simulink model "SOlar_panel_project"  (R2023b)
settings: Solver=FixedStepDiscrete  StartTime=0.0  StopTime=inf  FixedStep=1e-3  RelTol=1e-3
settings Model: ExtModeTrigDuration=2  Creator=Beshary  LastModifiedBy=Beshary
settings OptimizationCC: DefaultParameterBehavior=Inlined  UseDivisionForNetSlopeComputation=on  GainParamInheritBuiltInType=on  UseFloatMulNetSlope=on  InlineInvariantSignals=on  PassReuseOutputArgsAs=Individual arguments  ZeroExternalMemoryAtStartup=off  ZeroInternalMemoryAtStartup=off  NoFixptDivByZeroProtection=on  EfficientFloat2IntCast=on  LifeSpan=1  MaxStackSize=64  OptimizeBlockOrder=speed  DifferentSizesBufferReuse=on  EfficientTunableParamExpr=on
settings DebuggingCC: ParameterTunabilityLossMsg=error
settings HardwareCC: ProdBitPerInt=16  ProdBitPerPointer=16  ProdBitPerSizeT=16  ProdBitPerPtrDiffT=16  ProdLargestAtomicFloat=None  ProdWordSize=8  ProdLongLongMode=on  ProdHWDeviceType=Atmel->AVR
settings SFSimCC: MATLABDynamicMemAlloc=off
settings RTWCC: Description=Embedded Coder  SystemTargetFile=ert.tlc  HardwareBoard=Arduino Uno  TemplateMakefile=ert_default_tmf  Toolchain=Arduino AVR  BuildConfiguration=Faster Runs
settings CodeAppCC: ForceParamTrailComments=on  IgnoreCustomStorageClasses=off  OperatorAnnotations=on  SimulinkDataObjDesc=on  SFDataObjDesc=on  CustomSymbolStrGlobalVar=rt$N$M  CustomSymbolStrType=$N$M  CustomSymbolStrFcn=$N$M$F  CustomSymbolStrMacro=$N$M  InsertBlockDesc=on
settings ERTTargetCC: IncludeMdlTerminateFcn=off  CombineSignalStateStructs=on  SupportAbsoluteTime=off  SupportComplex=off  SupportNonInlinedSFcns=on  ExtModeTransport=3  ExtModeStaticAlloc=on  ExtModeAutomaticAllocSize=off  ExtModeStaticAllocSize=250  ExtModeMexFile=ext_xcp  ExtModeIntrfLevel=Level2 - Open  InlinedParameterPlacement=NonHierarchical  ERTFilePackagingFormat=CompactWithDataFile

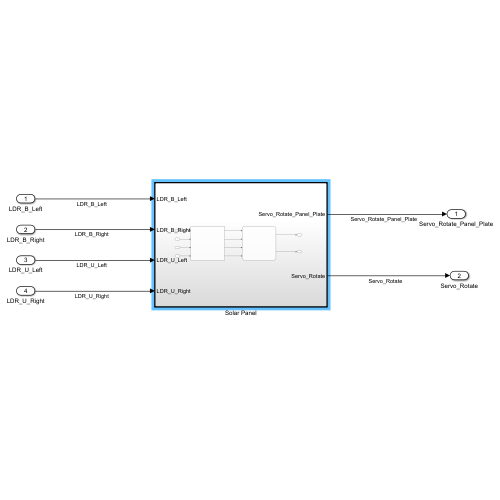
[thumbnail: Simulink's stored preview of the top-level diagram]
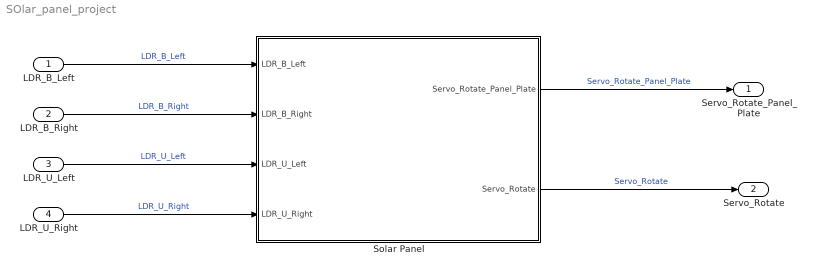
== system SOlar_panel_project ==
  LDR_B_Left : Inport
  LDR_B_Right : Inport  Port=2
  LDR_U_Left : Inport  Port=3
  LDR_U_Right : Inport  Port=4
  Solar Panel : Subsystem  TreatAsAtomicUnit=on
  Servo_Rotate_Panel_Plate : Outport
  Servo_Rotate : Outport  Port=2
  wires:
  LDR_B_Left/1 -> Solar Panel/1(LDR_B_Left)  "LDR_B_Left"
  LDR_B_Right/1 -> Solar Panel/2(LDR_B_Right)  "LDR_B_Right"
  LDR_U_Left/1 -> Solar Panel/3(LDR_U_Left)  "LDR_U_Left"
  LDR_U_Right/1 -> Solar Panel/4(LDR_U_Right)  "LDR_U_Right"
  Solar Panel/1(Servo_Rotate_Panel_Plate) -> Servo_Rotate_Panel_Plate/1  "Servo_Rotate_Panel_Plate"
  Solar Panel/2(Servo_Rotate) -> Servo_Rotate/1  "Servo_Rotate"

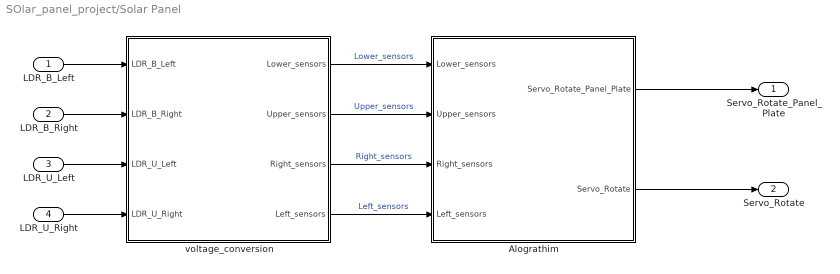
== system SOlar_panel_project/Solar Panel ==
  LDR_B_Left : Inport
  LDR_B_Right : Inport  Port=2
  LDR_U_Left : Inport  Port=3
  LDR_U_Right : Inport  Port=4
  "Alograthim " : Stateflow chart  TreatAsAtomicUnit=on
      settings: PortSchema="{\"entries\":[{\"content\":{\"sides\":[{\"content\":{\"connectorIds\":[\"In2\",\"In1\",\"In3\",\"In4\"]},\"type\":\"ConnectorPlacement.EquallySpacedRectSide\",\"uuid\":\"47346178-62f1-4af9-966f-6088c34d7d3a\"},{\"content\":{\"connectorIds\":[\"Out1\",\"Out2\"],\"side\":\"RIGHT\"},\"type\":\"ConnectorPlacement.EquallySpacedRectSide\",\"uuid\":\"d42f0d69-c7c6-440d-b039-ff859220b6c7\"},{\"content\":{\"side\":\"TOP\"},\"type\":\"ConnectorPlacement.EquallySpacedRectSide\",\"uuid\":\"40083903-8935-43d1-87ca-0c4b4a5851ce\"}]},\"type\":\"ConnectorPlacement.EquallySpacedConnector\",\"uuid\":\"c94df97a-4768-4a21-83be-24c93ffa522d\"}],\"packageUris\":[\"http://schema.mathworks.com/mf0/Connector/R2020b\"],\"version\":\"1.0\"}"
  voltage_conversion : Subsystem
  Servo_Rotate_Panel_Plate : Outport
  Servo_Rotate : Outport  Port=2
  wires:
  voltage_conversion/2(Upper_sensors) -> "Alograthim "/1(Upper_sensors)  "Upper_sensors"
  voltage_conversion/3(Right_sensors) -> "Alograthim "/3(Right_sensors)  "Right_sensors"
  LDR_B_Right/1 -> voltage_conversion/2(LDR_B_Right)
  "Alograthim "/2(Servo_Rotate) -> Servo_Rotate/1
  voltage_conversion/1(Lower_sensors) -> "Alograthim "/2(Lower_sensors)  "Lower_sensors"
  LDR_B_Left/1 -> voltage_conversion/1(LDR_B_Left)
  LDR_U_Left/1 -> voltage_conversion/3(LDR_U_Left)
  voltage_conversion/4(Left_sensors) -> "Alograthim "/4(Left_sensors)  "Left_sensors"
  "Alograthim "/1(Servo_Rotate_Panel_Plate) -> Servo_Rotate_Panel_Plate/1
  LDR_U_Right/1 -> voltage_conversion/4(LDR_U_Right)

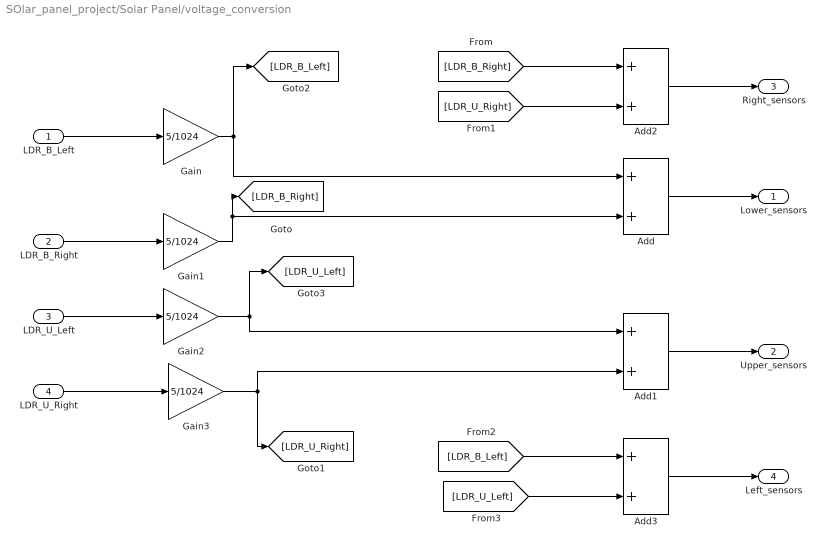
== system SOlar_panel_project/Solar Panel/voltage_conversion ==
  LDR_B_Left : Inport
  LDR_B_Right : Inport  Port=2
  LDR_U_Left : Inport  Port=3
  LDR_U_Right : Inport  Port=4
  Add{,1..3} (4 alike) : Sum
  Gain{,1..3} (4 alike) : Gain  Gain=5/1024
  Lower_sensors : Outport
  Upper_sensors : Outport  Port=2
  Right_sensors : Outport  Port=3
  Left_sensors : Outport  Port=4
  wires:
  LDR_U_Right/1 -> Gain3/1
  LDR_U_Left/1 -> Gain2/1
  LDR_B_Right/1 -> Gain1/1
  LDR_B_Left/1 -> Gain/1
  Gain3/1 -> [LDR_U_Right], Add1/2
  Gain/1 -> [LDR_B_Left], Add/1
  Gain1/1 -> [LDR_B_Right], Add/2
  Add/1 -> Lower_sensors/1
  Add1/1 -> Upper_sensors/1
  [LDR_B_Right] -> Add2/1
  [LDR_U_Right] -> Add2/2
  Add2/1 -> Right_sensors/1
  [LDR_B_Left] -> Add3/1
  Add3/1 -> Left_sensors/1
  [LDR_U_Left] -> Add3/2
  Gain2/1 -> [LDR_U_Left], Add1/1

== stateflow chart SOlar_panel_project/Solar Panel/Alograthim  ==
  state Servo_land [parallel]
    en:
    du:
    Servo_Rotate=servo_land(Right_sensors,Left_sensors);
    settings: executionOrder=1
  state servo_panel1 [parallel]
    en:
    du:
    Servo_Rotate_Panel_Plate=servo_panel(Upper_sensors,Lower_sensors);
    settings: executionOrder=2
  state Servo_out=servo_panel(Upper_sensors,Lower_sensors) [function]
    (default) -> (junction 107) : /* speed */
    (junction 107) -> (junction 124) [order 1] : [abs(Upper_sensors-Lower_sensors)<=0.5]
    (junction 107) -> (junction 116) [order 2]
    (junction 124) -> (junction 114) : {Servo_out=0;}
    (junction 116) -> (junction 115) [order 1] : [Upper_sensors>Lower_sensors]
    (junction 116) -> (junction 111) [order 2] : {Servo_out=(Upper_sensors/2)*(255/5)*Step_angle;}
    (junction 115) -> (junction 123) : {Servo_out=(Lower_sensors/2)*(255/5)*Step_angle;}
    (junction 123) -> (junction 111)
    (junction 114) -> (junction 123)
    (junction 111) -> (junction 110)
  state Servo_out_land=servo_land(Right_sensors,Left_sensors) [function]
    (default) -> (junction 99) : /* speed */
    (junction 99) -> (junction 100) [order 1] : [abs(Right_sensors-Left_sensors)<=0.5]
    (junction 99) -> (junction 101) [order 2]
    (junction 100) -> (junction 105) : {Servo_out_land=0;}
    (junction 101) -> (junction 102) [order 1] : [Right_sensors>Left_sensors]
    (junction 101) -> (junction 103) [order 2] : {Servo_out_land=(Right_sensors/2)*(255/5)*Step_angle;}
    (junction 102) -> (junction 104) : {Servo_out_land=(Left_sensors/2)*(255/5)*Step_angle;}
    (junction 104) -> (junction 103)
    (junction 105) -> (junction 104)
    (junction 103) -> (junction 106)
  data: Servo_out function_output double; Upper_sensors function_input double; Lower_sensors function_input double; Servo_out_land function_output double; Right_sensors function_input double; Left_sensors function_input double; Servo_Rotate_Panel_Plate output; Upper_sensors input; Lower_sensors input; Right_sensors input; Left_sensors input; Servo_Rotate output; Step_angle local double =180/255
